simulink model "controller"  (R2021a)
settings: Solver=VariableStepAuto  StartTime=0  StopTime=100  RelTol=1e-3
libraries: pid_lib x2, simulink x1
settings Model: Creator=admin  LastModifiedBy=admin
settings DataIOCC: SaveFormat=StructureWithTime
settings OptimizationCC: BlockReduction=off  BufferReuse=off
settings DebuggingCC: AlgebraicLoopMsg=none  UnconnectedInputMsg=none  UnconnectedOutputMsg=none  UnconnectedLineMsg=none

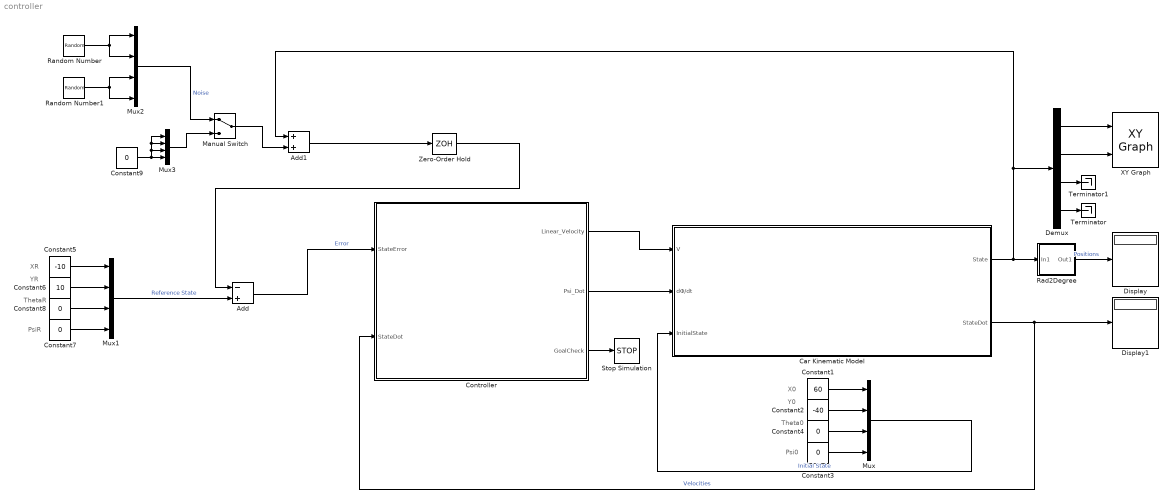
== system controller ==
  note: Psi0
  note: Y0
  note: Theta0
  note: X0
  note: XR
  note: YR
  note: PsiR
  note: ThetaR
  Add : Sum  Inputs=-+
  Add1 : Sum
  Car Kinematic Model : Subsystem
  Constant1 : Constant  Value=60  SampleTime=0.001
  Constant2 : Constant  Value=-40  SampleTime=0.001
  Constant{3..4,7..9} (5 alike) : Constant  Value=0  SampleTime=0.001
  Constant5 : Constant  Value=-10  SampleTime=0.001
  Constant6 : Constant  Value=10  SampleTime=0.001
  Controller : Subsystem
  Demux : Demux
  Display : Display
  Display1 : Display
  Manual Switch : ManualSwitch
  Mux{,1..3} (4 alike) : Mux
  Rad2Degree : Subsystem
  Random Number : RandomNumber  Variance=0.005  SampleTime=0.001
  Random Number1 : RandomNumber  Variance=0.002  SampleTime=0.001
  Stop Simulation : Stop
  Terminator : Terminator
  Terminator1 : Terminator
  XY Graph : simulink/Sinks/XY Graph  xmin=-100  xmax=100  ymin=-100  ymax=100  st=0.001
  Zero-Order Hold : ZeroOrderHold  SampleTime=0.001
  wires:
  Constant3/1 -> Mux/4
  Constant1/1 -> Mux/1
  Constant2/1 -> Mux/2
  Constant4/1 -> Mux/3
  Mux/1 -> Car Kinematic Model/3(InitialState)  "Initial State"
  Car Kinematic Model/1(State) -> Rad2Degree/1(In1), Demux/1, Add1/1
  Car Kinematic Model/2(StateDot) -> Controller/2(StateDot), Display1/1  "Velocities"
  Constant8/1 -> Mux1/3
  Constant7/1 -> Mux1/4
  Constant5/1 -> Mux1/1
  Constant6/1 -> Mux1/2
  Controller/2(Psi_Dot) -> Car Kinematic Model/2(dΦ/dt)
  Controller/1(Linear_Velocity) -> Car Kinematic Model/1(V)
  Add/1 -> Controller/1(StateError)  "Error"
  Mux1/1 -> Add/2  "Reference State"
  Demux/2 -> XY Graph/2
  Demux/1 -> XY Graph/1
  Demux/3 -> Terminator1/1
  Demux/4 -> Terminator/1
  Mux2/1 -> Manual Switch/1  "Noise"
  Add1/1 -> Zero-Order Hold/1
  Random Number/1 -> Mux2/1, Mux2/2
  Random Number1/1 -> Mux2/4, Mux2/3
  Manual Switch/1 -> Add1/2
  Mux3/1 -> Manual Switch/2
  Constant9/1 -> Mux3/2, Mux3/1, Mux3/3, Mux3/4
  Controller/3(GoalCheck) -> Stop Simulation/1
  Rad2Degree/1(Out1) -> Display/1  "Positions"
  Zero-Order Hold/1 -> Add/1

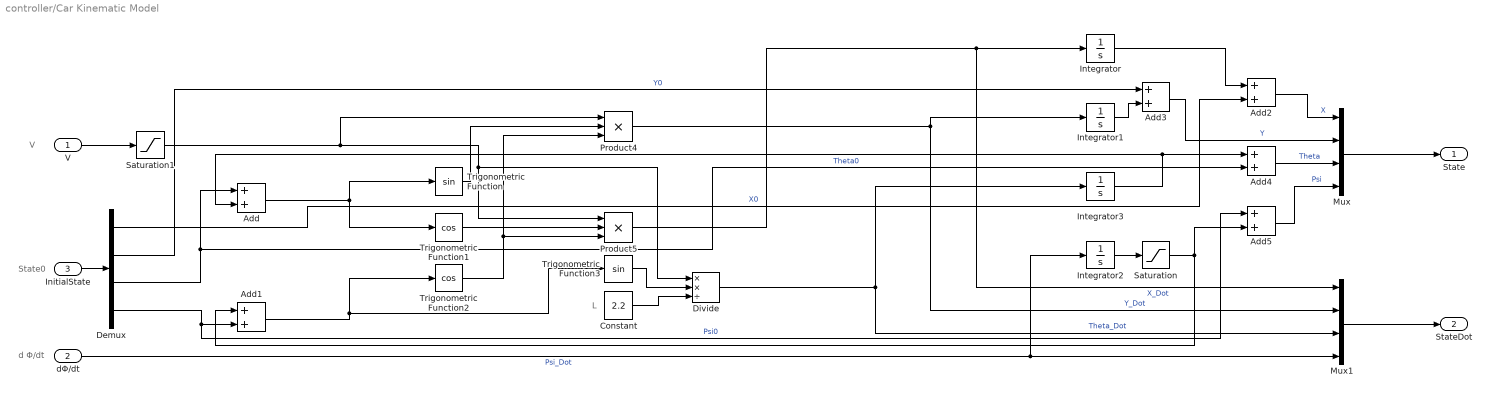
== system controller/Car Kinematic Model ==
  note: d Φ/dt
  note: V
  note: L
  note: State0
  V : Inport
  dΦ/dt : Inport  Port=2
  InitialState : Inport  Port=3
  Add{,1..5} (6 alike) : Sum
  Constant : Constant  Value=2.2
  Demux : Demux
  Divide : Product  Inputs=**/
  Integrator{,1..3} (4 alike) : Integrator
  Mux : Mux
  Mux1 : Mux
  Product4 : Product  Inputs=3
  Product5 : Product  Inputs=3
  Saturation : Saturate  UpperLimit=pi/4  LowerLimit=-pi/4
  Saturation1 : Saturate  UpperLimit=5.556  LowerLimit=-5.556
  Trigonometric Function : Trigonometry
  Trigonometric Function1 : Trigonometry  Operator=cos
  Trigonometric Function2 : Trigonometry  Operator=cos
  Trigonometric Function3 : Trigonometry  OutputSignalType=real
  State : Outport
  StateDot : Outport  Port=2
  wires:
  Mux/1 -> State/1
  Mux1/1 -> StateDot/1
  V/1 -> Saturation1/1
  Trigonometric Function/1 -> Product4/2
  Trigonometric Function2/1 -> Product5/3, Product4/3
  Trigonometric Function1/1 -> Product5/2
  Trigonometric Function3/1 -> Divide/2
  Constant/1 -> Divide/3
  dΦ/dt/1 -> Integrator2/1, Mux1/4  "Psi_Dot"
  Demux/3 -> Add4/2, Add/1  "Theta0"
  Demux/4 -> Add1/2, Add5/1  "Psi0"
  Add/1 -> Trigonometric Function1/1, Trigonometric Function/1
  Add1/1 -> Trigonometric Function3/1, Trigonometric Function2/1
  Integrator2/1 -> Saturation/1
  Divide/1 -> Mux1/3, Integrator3/1  "Theta_Dot"
  Integrator3/1 -> Add4/1, Add/2
  Product5/1 -> Mux1/1, Integrator/1  "X_Dot"
  Integrator/1 -> Add2/1
  Product4/1 -> Integrator1/1, Mux1/2  "Y_Dot"
  InitialState/1 -> Demux/1
  Demux/1 -> Add2/2  "X0"
  Demux/2 -> Add3/1  "Y0"
  Add2/1 -> Mux/1  "X"
  Integrator1/1 -> Add3/2
  Add3/1 -> Mux/2  "Y"
  Saturation/1 -> Add5/2, Add1/1
  Add4/1 -> Mux/3  "Theta"
  Add5/1 -> Mux/4  "Psi"
  Saturation1/1 -> Divide/1, Product5/1, Product4/1

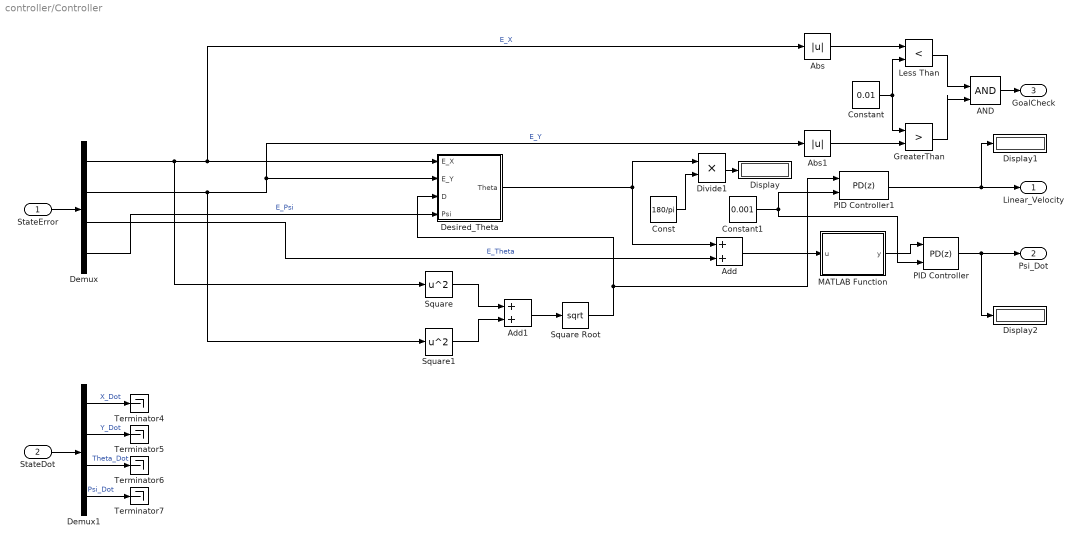
== system controller/Controller ==
  StateError : Inport
  StateDot : Inport  Port=2
  AND : Logic  IconShape=distinctive  AllPortsSameDT=off  OutDataTypeStr=boolean
  Abs : Abs
  Abs1 : Abs
  Add : Sum
  Add1 : Sum
  Const : Constant  Value=180/pi
  Constant : Constant  Value=0.01
  Constant1 : Constant  Value=0.001  SampleTime=0.001
  Demux : Demux
  Demux1 : Demux
  Desired_Theta : Subsystem
  Display : Display
  Display1 : Display
  Display2 : Display
  Divide1 : Product  Inputs=**
  GreaterThan : RelationalOperator  Operator=>  OutDataTypeStr=boolean  RndMeth=Simplest
  Less Than : RelationalOperator  Operator=<  OutDataTypeStr=boolean  RndMeth=Simplest
  MATLAB Function : MATLAB Function  TreatAsAtomicUnit=on
  PID Controller : pid_lib/PID Controller  Controller=PD  Form=Parallel  TimeDomain=Discrete-time  UseExternalTs=on  SampleTime=-1  IntegratorMethod=Forward Euler  FilterMethod=Forward Euler  ControllerParametersSource=internal  P=8.5  I=3.85  D=4.5  UseFilter=on  N=65  TunerSelectOption=Transfer Function Based (PID Tuner App)  InitialConditionSource=internal  InitialConditionForIntegrator=0  InitialConditionForFilter=0  DifferentiatorICPrevScaledInput=0  ExternalReset=none  TrackingMode=off  Kt=1  LimitOutput=off  SatLimitsSource=internal  UpperSaturationLimit=inf  LowerSaturationLimit=-inf  LinearizeAsGain=on  AntiWindupMode=none  Kb=1  POutMin=[]  POutMax=[]  IOutMin=[]  IOutMax=[]  DOutMin=[]  DOutMax=[]  NOutMin=[]  NOutMax=[]  SumOutMin=[]  SumOutMax=[]  SaturationOutMin=[]  SaturationOutMax=[]  PParamMin=[]  PParamMax=[]  IParamMin=[]  IParamMax=[]  DParamMin=[]  DParamMax=[]  NParamMin=[]  NParamMax=[]  KbParamMin=[]  KbParamMax=[]  KtParamMin=[]  KtParamMax=[]  KbOutMin=[]  KbOutMax=[]  KtOutMin=[]  KtOutMax=[]  IntegratorOutMin=[]  IntegratorOutMax=[]  FilterOutMin=[]  FilterOutMax=[]  SumI1OutMin=[]  SumI1OutMax=[]  SumI2OutMin=[]  SumI2OutMax=[]  SumI3OutMin=[]  SumI3OutMax=[]  SumI4OutMin=[]  SumI4OutMax=[]  SumDOutMin=[]  SumDOutMax=[]  DifferentiatorOutMin=[]  DifferentiatorOutMax=[]  FilterDiffOutCoefMin=[]  FilterDiffOutCoefMax=[]  ReciprocalOutMin=[]  ReciprocalOutMax=[]  SumDenOutMin=[]  SumDenOutMax=[]  SumNumOutMin=[]  SumNumOutMax=[]  DivideOutMin=[]  DivideOutMax=[]  UdiffTsProdOutMin=[]  UdiffTsProdOutMax=[]  NTsProdOutMin=[]  NTsProdOutMax=[]  UintegralTsProdOutMin=[]  UintegralTsProdOutMax=[]  UngainTsProdOutMin=[]  UngainTsProdOutMax=[]  IntegratorContinuousStateAttributes=''  IntegratorStateMustResolveToSignalObject=off  IntegratorRTWStateStorageClass=Auto  FilterContinuousStateAttributes=''  FilterStateMustResolveToSignalObject=off  FilterRTWStateStorageClass=Auto  ParallelPVariant=InternalParameters  IdealPVariant=Disabled  IVariant=Disabled  DVariant=InternalParameters  IntegratorVariant=Disabled  SatVariant=Disabled  AWVariant=Disabled  PCopyVariant=Disabled  TRVariant=Disabled  FdbkBlocksVariant=Forward  IdealPFdbkVariant=Disabled  SatFdbkVariant=Disabled  DerivativeFilterVariant=ForwardEulerFilter  NVariant=InternalParameters  NCopyVariant=Disabled  FilterICVariant=InternalICsFilter  IntegratorICVariant=Disabled  ExternalResetVariant=Disabled  TRSumVariant=Passthrough  SumFdbkVariant=Disabled  SumVariant=Sum_PD  TsampFilterVariant=ExternalTs  TsampNgainVariant=ExternalTs  TsampIntegralVariant=Disabled  ExternalSaturationOutDataTypeStr=Inherit: Same as second input
  PID Controller1 : pid_lib/PID Controller  Controller=PD  Form=Parallel  TimeDomain=Discrete-time  UseExternalTs=on  SampleTime=0.001  IntegratorMethod=Forward Euler  FilterMethod=Forward Euler  ControllerParametersSource=internal  P=4  I=0.001  D=8  UseFilter=on  N=4  TunerSelectOption=Transfer Function Based (PID Tuner App)  InitialConditionSource=internal  InitialConditionForIntegrator=0  InitialConditionForFilter=0  DifferentiatorICPrevScaledInput=0  ExternalReset=none  TrackingMode=off  Kt=1  LimitOutput=off  SatLimitsSource=internal  UpperSaturationLimit=inf  LowerSaturationLimit=-inf  LinearizeAsGain=on  AntiWindupMode=none  Kb=1  POutMin=[]  POutMax=[]  IOutMin=[]  IOutMax=[]  DOutMin=[]  DOutMax=[]  NOutMin=[]  NOutMax=[]  SumOutMin=[]  SumOutMax=[]  SaturationOutMin=[]  SaturationOutMax=[]  PParamMin=[]  PParamMax=[]  IParamMin=[]  IParamMax=[]  DParamMin=[]  DParamMax=[]  NParamMin=[]  NParamMax=[]  KbParamMin=[]  KbParamMax=[]  KtParamMin=[]  KtParamMax=[]  KbOutMin=[]  KbOutMax=[]  KtOutMin=[]  KtOutMax=[]  IntegratorOutMin=[]  IntegratorOutMax=[]  FilterOutMin=[]  FilterOutMax=[]  SumI1OutMin=[]  SumI1OutMax=[]  SumI2OutMin=[]  SumI2OutMax=[]  SumI3OutMin=[]  SumI3OutMax=[]  SumI4OutMin=[]  SumI4OutMax=[]  SumDOutMin=[]  SumDOutMax=[]  DifferentiatorOutMin=[]  DifferentiatorOutMax=[]  FilterDiffOutCoefMin=[]  FilterDiffOutCoefMax=[]  ReciprocalOutMin=[]  ReciprocalOutMax=[]  SumDenOutMin=[]  SumDenOutMax=[]  SumNumOutMin=[]  SumNumOutMax=[]  DivideOutMin=[]  DivideOutMax=[]  UdiffTsProdOutMin=[]  UdiffTsProdOutMax=[]  NTsProdOutMin=[]  NTsProdOutMax=[]  UintegralTsProdOutMin=[]  UintegralTsProdOutMax=[]  UngainTsProdOutMin=[]  UngainTsProdOutMax=[]  IntegratorContinuousStateAttributes=''  IntegratorStateMustResolveToSignalObject=off  IntegratorRTWStateStorageClass=Auto  FilterContinuousStateAttributes=''  FilterStateMustResolveToSignalObject=off  FilterRTWStateStorageClass=Auto  ParallelPVariant=InternalParameters  IdealPVariant=Disabled  IVariant=Disabled  DVariant=InternalParameters  IntegratorVariant=Disabled  SatVariant=Disabled  AWVariant=Disabled  PCopyVariant=Disabled  TRVariant=Disabled  FdbkBlocksVariant=Forward  IdealPFdbkVariant=Disabled  SatFdbkVariant=Disabled  DerivativeFilterVariant=ForwardEulerFilter  NVariant=InternalParameters  NCopyVariant=Disabled  FilterICVariant=InternalICsFilter  IntegratorICVariant=Disabled  ExternalResetVariant=Disabled  TRSumVariant=Passthrough  SumFdbkVariant=Disabled  SumVariant=Sum_PD  TsampFilterVariant=ExternalTs  TsampNgainVariant=ExternalTs  TsampIntegralVariant=Disabled  ExternalSaturationOutDataTypeStr=Inherit: Same as second input
  Square : Math  Operator=square  SaturateOnIntegerOverflow=on
  Square Root : Sqrt  SaturateOnIntegerOverflow=on
  Square1 : Math  Operator=square  SaturateOnIntegerOverflow=on
  Terminator{4..7} (4 alike) : Terminator
  Linear_Velocity : Outport
  Psi_Dot : Outport  Port=2
  GoalCheck : Outport  Port=3
  wires:
  StateError/1 -> Demux/1
  Demux/2 -> Square1/1, Abs1/1, Desired_Theta/2(E_Y)  "E_Y"
  Demux/3 -> Add/2  "E_Theta"
  PID Controller/1 -> Display2/1, Psi_Dot/1
  StateDot/1 -> Demux1/1
  Demux1/1 -> Terminator4/1  "X_Dot"
  Demux1/4 -> Terminator7/1  "Psi_Dot"
  Demux1/3 -> Terminator6/1  "Theta_Dot"
  Demux1/2 -> Terminator5/1  "Y_Dot"
  Demux/1 -> Square/1, Abs/1, Desired_Theta/1(E_X)  "E_X"
  Demux/4 -> Desired_Theta/4(Psi)  "E_Psi"
  PID Controller1/1 -> Display1/1, Linear_Velocity/1
  Constant/1 -> GreaterThan/1, Less Than/2
  Less Than/1 -> AND/1
  GreaterThan/1 -> AND/2
  AND/1 -> GoalCheck/1
  Square/1 -> Add1/1
  Square1/1 -> Add1/2
  Add1/1 -> Square Root/1
  Square Root/1 -> PID Controller1/1, Desired_Theta/3(D)
  Add/1 -> MATLAB Function/1(u)
  Const/1 -> Divide1/2
  Divide1/1 -> Display/1
  Desired_Theta/1(Theta) -> Divide1/1, Add/1
  Abs/1 -> Less Than/1
  Abs1/1 -> GreaterThan/2
  MATLAB Function/1(y) -> PID Controller/1
  Constant1/1 -> PID Controller/2, PID Controller1/2

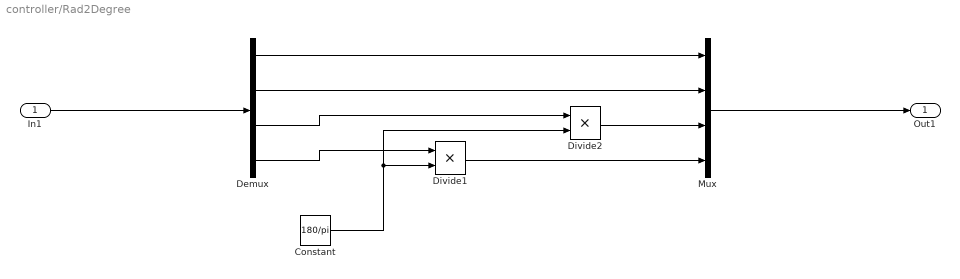
== system controller/Rad2Degree ==
  In1 : Inport
  Constant : Constant  Value=180/pi
  Demux : Demux
  Divide1 : Product  Inputs=**
  Divide2 : Product  Inputs=**
  Mux : Mux
  Out1 : Outport
  wires:
  In1/1 -> Demux/1
  Mux/1 -> Out1/1
  Demux/1 -> Mux/1
  Demux/2 -> Mux/2
  Demux/3 -> Divide2/1
  Demux/4 -> Divide1/1
  Constant/1 -> Divide1/2, Divide2/2
  Divide1/1 -> Mux/4
  Divide2/1 -> Mux/3

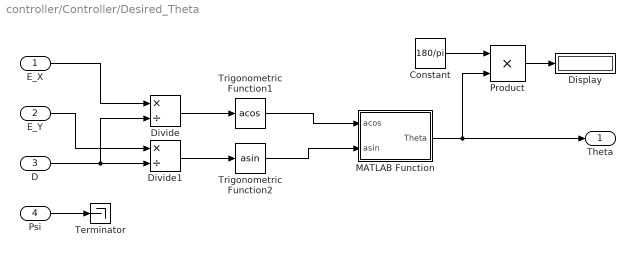
== system controller/Controller/Desired_Theta ==
  E_X : Inport
  E_Y : Inport  Port=2
  D : Inport  Port=3
  Psi : Inport  Port=4
  Constant : Constant  Value=180/pi
  Display : Display
  Divide : Product  Inputs=*/
  Divide1 : Product  Inputs=*/
  MATLAB Function : MATLAB Function  TreatAsAtomicUnit=on
  Product : Product
  Terminator : Terminator
  Trigonometric Function1 : Trigonometry  Operator=acos
  Trigonometric Function2 : Trigonometry  Operator=asin
  Theta : Outport
  wires:
  D/1 -> Divide/2, Divide1/2
  E_X/1 -> Divide/1
  Divide/1 -> Trigonometric Function1/1
  E_Y/1 -> Divide1/1
  Divide1/1 -> Trigonometric Function2/1
  Psi/1 -> Terminator/1
  Trigonometric Function2/1 -> MATLAB Function/2(asin)
  Trigonometric Function1/1 -> MATLAB Function/1(acos)
  MATLAB Function/1(Theta) -> Theta/1, Product/2
  Constant/1 -> Product/1
  Product/1 -> Display/1

== matlab function controller/Controller/Desired_Theta/MATLAB Function ==
  data: acos input; Theta output; asin input
function Theta = fcn(acos, asin)
if acos==asin
    K = acos;
elseif (acos > pi/2) && (asin > 0)
    K = acos;
elseif (acos > pi/2) && (asin < 0)
    K = -pi-asin;
else
    K = asin;
end    
Theta = K;

== matlab function controller/Controller/MATLAB Function ==
  data: u input; y output
function y = fcn(u)
if u>0
    if u > pi
        K = u-2*pi;
    else
        K = u;
    end
else
    if u < -pi
        K = 2*pi+u;
    else
        K = u;
    end
end
y = K;
